simulink model "cranebot_cable"  (R2020b)
settings: Solver=ode15s  StartTime=0.0  StopTime=T  MaxStep=0.01  RelTol=1e-3
values from neighbouring files (symbols this model uses):
  friction = [fv1p fv2p fv1 fv2 fv3 fv4 fv5 fv6 fv1 fv2 fv3 fv4 fv5 fv6]    [sim_cranebot_cable.m]
  g = [0 0 -g0]'    [sim_cranebot_cable.m]
  info = struct('n_joints', n_joints,                'n_links', n_links,                'n_ee', n_ee,                'current_frame_index',  [ 1  2 3 4 5 6 7  8  9 10 11 12 13 14 15 16],                'previous_frame_index', [ 0  1 2 3 4 5 6  7  2  9 10 11 12 13  8 14],               'next_frame_index',     [ 2 39 4 5 6 7 8 15 10 11 12 13 14 16  0  0],               'next_frame_type',      [ 0  1 0 0 0 0  ...(+639 chars)    [sim_cranebot_cable.m]
  Kd = 10*eye(12)    [sim_cranebot_cable.m]
  Kp = 10*eye(12)    [sim_cranebot_cable.m]
  q_ref = [-pi/8 -pi/8 pi/4 -pi/4 0 0 -pi/8 -pi/8 pi/4 -pi/4 0 0]'    [sim_cranebot_cable.m]
  qd_ref = zeros(1,12)    [sim_cranebot_cable.m]
  qdd_ref = zeros(1,12)    [sim_cranebot_cable.m]
  th1A_0 = deg2rad(0)    [sim_cranebot_cable.m]
  th1B_0 = deg2rad(0)    [sim_cranebot_cable.m]
  th2A_0 = deg2rad(0)    [sim_cranebot_cable.m]
  th2B_0 = deg2rad(0)    [sim_cranebot_cable.m]
  th3A_0 = deg2rad(0)    [sim_cranebot_cable.m]
  th3B_0 = deg2rad(0)    [sim_cranebot_cable.m]
  th4A_0 = deg2rad(0)    [sim_cranebot_cable.m]
  th4B_0 = deg2rad(0)    [sim_cranebot_cable.m]
  th5A_0 = deg2rad(0)    [sim_cranebot_cable.m]
  th5B_0 = deg2rad(0)    [sim_cranebot_cable.m]
  th6A_0 = deg2rad(0)    [sim_cranebot_cable.m]
  th6B_0 = deg2rad(0)    [sim_cranebot_cable.m]
undefined symbols (not defined in the file or in its folder): D, ixx_1, ixx_2, ixx_3, ixx_4, ixx_5, ixx_6, ixx_cables, ixx_platform, ixy_1, ixy_2, ixy_3, ixy_4, ixy_5, ixy_6, ixy_cables, ixy_platform, ixz_1, ixz_2, ixz_3, ixz_4, ixz_5, ixz_6, ixz_cables, ixz_platform, iyy_1, iyy_2, iyy_3, iyy_4, iyy_5, iyy_6, iyy_cables, iyy_platform, iyz_1, iyz_2, iyz_3, iyz_4, iyz_5, iyz_6, iyz_cables, iyz_platform, izz_1, izz_2, izz_3, izz_4, izz_5, izz_6, izz_cables, izz_platform, L, m_cables, m_crane, m_platform, ml1, ml2, ml3, ml4, ml5, ml6, offA ... (+4)
libraries: sm_lib x155, nesl_utility x58
(part 4 of 4)

== system cranebot_cable/Full system/Schunk Powerball B/link4 ==
  Inertia : sm_lib/Body Elements/Inertia  InertiaType=Custom  Mass=ml4  MassUnits=kg  CenterOfMass=[0, 0, 0]  CenterOfMassUnits=m  MomentsOfInertia=[ixx_4, iyy_4, izz_4]  MomentsOfInertiaUnits=kg*m^2  ProductsOfInertia=[iyz_4, ixz_4, ixy_4]  ProductsOfInertiaUnits=kg*m^2  GraphicType=None  MarkerShape=Inertia  MarkerSize=20  GraphicVisPropType=SimpleVisualProperties  GraphicDiffuseColor=[0.5 0.5 0.5]  GraphicSpecularColor=[0.5 0.5 0.5 1.0]  GraphicAmbientColor=[0.15 0.15 0.15 1.0]  GraphicEmissiveColor=[0.0 0.0 0.0 1.0]  GraphicShininess=75  GraphicOpacity=1.0
  InertiaOriginTransform : sm_lib/Frames and Transforms/Rigid Transform  TranslationMethod=Cartesian  TranslationStandardOffset=0  TranslationLengthUnit=m  TranslationStandardAxis=+Z  TranslationCartesianOffset=inertial_disp_4  TranslationROffset=0  TranslationROffsetUnits=m  TranslationZOffset=0  TranslationZOffsetUnits=m  TranslationThetaOffset=0  TranslationThetaOffsetUnits=deg  RotationMethod=RotationSequence  RotationAngleUnits=deg  RotationStandardAxis=+Z  RotationAngle=0.0  RotationArbitraryAxis=[0 0 1]  FollAlignAxisA=+X  BaseAlignAxisA=+Y  FollAlignAxisB=+Y  BaseAlignAxisB=+Z  RotationSequenceAxes=BaseAxes  RotationSequence=XYZ  RotationSequenceAngles=[0, 0, 0]  RotationSequenceAnglesUnits=rad  RotationMatrix=[1 0 0; 0 1 0; 0 0 1]
  ReferenceFrame : sm_lib/Frames and Transforms/Reference Frame
  Visual : sm_lib/Body Elements/File Solid  ExtGeomFileName=link4.stl  UnitType=Custom  ExtGeomFileUnits=m  StepReaderType=HEX  ExportConvexHullGeometry=off  InertiaType=Custom  Mass=0  MassUnits=kg  CenterOfMass=[0, 0, 0]  CenterOfMassUnits=m  MomentsOfInertia=[0, 0, 0]  MomentsOfInertiaUnits=kg*m^2  ProductsOfInertia=[0, 0, 0]  ProductsOfInertiaUnits=kg*m^2  BasedOnType=DensityFromFile  Density=1000  DensityUnits=kg/m^3  DoExposeReferenceFrame=on  SerializedFrames=<Frames/>  GraphicType=FromGeometry  MarkerShape=Sphere  MarkerSize=10  GraphicVisPropType=SimpleVisualProperties  GraphicDiffuseColor=[0, 0, 0.6]  GraphicSpecularColor=[0.5 0.5 0.5 1.0]  GraphicAmbientColor=[0.15 0.15 0.15 1.0]  GraphicEmissiveColor=[0.0 0.0 0.0 1.0]  GraphicShininess=75  GraphicOpacity=1
  VisualOriginTransform : sm_lib/Frames and Transforms/Rigid Transform  TranslationMethod=Cartesian  TranslationStandardOffset=0  TranslationLengthUnit=m  TranslationStandardAxis=+Z  TranslationCartesianOffset=[0, 0, 0]  TranslationROffset=0  TranslationROffsetUnits=m  TranslationZOffset=0  TranslationZOffsetUnits=m  TranslationThetaOffset=0  TranslationThetaOffsetUnits=deg  RotationMethod=RotationSequence  RotationAngleUnits=deg  RotationStandardAxis=+Z  RotationAngle=0.0  RotationArbitraryAxis=[0 0 1]  FollAlignAxisA=+X  BaseAlignAxisA=+Y  FollAlignAxisB=+Y  BaseAlignAxisB=+Z  RotationSequenceAxes=BaseAxes  RotationSequence=XYZ  RotationSequenceAngles=[0, 0, 0]  RotationSequenceAnglesUnits=rad  RotationMatrix=[1 0 0; 0 1 0; 0 0 1]
  erb145_link4_joint_AxisInvTransform : sm_lib/Frames and Transforms/Rigid Transform  TranslationMethod=Cartesian  TranslationStandardOffset=0  TranslationLengthUnit=m  TranslationStandardAxis=+Z  TranslationCartesianOffset=[0, 0, 0]  TranslationROffset=0  TranslationROffsetUnits=m  TranslationZOffset=0  TranslationZOffsetUnits=m  TranslationThetaOffset=0  TranslationThetaOffsetUnits=deg  RotationMethod=ArbitraryAxis  RotationAngleUnits=rad  RotationStandardAxis=+Z  RotationAngle=0  RotationArbitraryAxis=[1, 0, 0]  FollAlignAxisA=+X  BaseAlignAxisA=+Y  FollAlignAxisB=+Y  BaseAlignAxisB=+Z  RotationSequenceAxes=FollowerAxes  RotationSequence=XYX  RotationSequenceAngles=[0 0 0]  RotationSequenceAnglesUnits=deg  RotationMatrix=[1 0 0; 0 1 0; 0 0 1]
  link4_erb115_joint_AxisTransform : sm_lib/Frames and Transforms/Rigid Transform  TranslationMethod=Cartesian  TranslationStandardOffset=0  TranslationLengthUnit=m  TranslationStandardAxis=+Z  TranslationCartesianOffset=[0, 0, 0]  TranslationROffset=0  TranslationROffsetUnits=m  TranslationZOffset=0  TranslationZOffsetUnits=m  TranslationThetaOffset=0  TranslationThetaOffsetUnits=deg  RotationMethod=ArbitraryAxis  RotationAngleUnits=rad  RotationStandardAxis=+Z  RotationAngle=0  RotationArbitraryAxis=[1, 0, 0]  FollAlignAxisA=+X  BaseAlignAxisA=+Y  FollAlignAxisB=+Y  BaseAlignAxisB=+Z  RotationSequenceAxes=FollowerAxes  RotationSequence=XYX  RotationSequenceAngles=[0 0 0]  RotationSequenceAnglesUnits=deg  RotationMatrix=[1 0 0; 0 1 0; 0 0 1]
  link4_erb115_joint_OriginTransform : sm_lib/Frames and Transforms/Rigid Transform  TranslationMethod=Cartesian  TranslationStandardOffset=0  TranslationLengthUnit=m  TranslationStandardAxis=+Z  TranslationCartesianOffset=[0, 0, 0.305]  TranslationROffset=0  TranslationROffsetUnits=m  TranslationZOffset=0  TranslationZOffsetUnits=m  TranslationThetaOffset=0  TranslationThetaOffsetUnits=deg  RotationMethod=RotationSequence  RotationAngleUnits=deg  RotationStandardAxis=+Z  RotationAngle=0.0  RotationArbitraryAxis=[0 0 1]  FollAlignAxisA=+X  BaseAlignAxisA=+Y  FollAlignAxisB=+Y  BaseAlignAxisB=+Z  RotationSequenceAxes=BaseAxes  RotationSequence=XYZ  RotationSequenceAngles=[-1.57079632675, 0, 0]  RotationSequenceAnglesUnits=rad  RotationMatrix=[1 0 0; 0 1 0; 0 0 1]
  F : PMIOPort  Side=Left
  F1 : PMIOPort  Port=2  Side=Right
  connections:
  Inertia/RConn1 -- InertiaOriginTransform/RConn1
  erb145_link4_joint_AxisInvTransform/LConn1 -- link4_erb115_joint_OriginTransform/LConn1 -- ReferenceFrame/RConn1 -- InertiaOriginTransform/LConn1 -- VisualOriginTransform/LConn1
  Visual/RConn1 -- VisualOriginTransform/RConn1
  erb145_link4_joint_AxisInvTransform/RConn1 -- F/RConn1
  link4_erb115_joint_AxisTransform/RConn1 -- F1/RConn1
  link4_erb115_joint_AxisTransform/LConn1 -- link4_erb115_joint_OriginTransform/RConn1

== matlab function cranebot_cable/MATLAB Function1 ==
  data: q input; qd input; qd_att output; q_att output
function [qd_att, q_att] = fcn(q, qd)

qd_att = qd(3:14);
q_att = q(3:14);

end

== matlab function cranebot_cable/Partial FBL (cable) ==
  data: y input; theta input; dtheta input; g parameter; tau output; info parameter; friction parameter
function tau = fcn(y, theta, dtheta, g, info, friction)

    n_joints = 14;

    % Computation B matrix
    B = zeros(n_joints,n_joints);
    for i=1:n_joints
        fake_acc = zeros(1,n_joints);
        fake_acc(i) = 1;
        B(:,i) = recursive_invdyn_tree_f(theta, zeros(1,n_joints), fake_acc, zeros(3,1), info);
    end
    
    % Computation n vector
    Fv = diag([friction(1), friction(2), friction(3), friction(4), friction(5), friction(6), friction(7), friction(8), friction(9), friction(10), friction(11), friction(12), friction(13), friction(14)]);
    n = recursive_invdyn_tree_f(theta, dtheta, zeros(1,n_joints), g, info) + Fv*dtheta;
   
    % Partial Feedback Linearization
    Bm = B(3:14,3:14);
    Bmb = B(3:14,1:2);
    Bbm = B(1:2,3:14);
    Bb = B(1:2,1:2);
    nb = n(1:2);
    nm = n(3:14);

    B_tilde = (Bm-Bmb*inv(Bb)*Bbm);
    n_tilde = nm - Bmb*inv(Bb)*nb;

    tau = B_tilde*y + n_tilde;
    
end
